simulink model "draft_arm_model"  (R2021b)
settings: Solver=VariableStepAuto  StartTime=0.0  StopTime=8  RelTol=1e-3
values from neighbouring files (symbols this model uses):
  gear_i = 2    [draft_model_variables.m]    (also in linear_model_variables.m = 1)
  ka = km    (= 0.0228)    [draft_model_variables.m]    (also in linear_model_variables.m = 0.0849)
  Kd = 2    [draft_model_variables.m]
  Ki = 0    [draft_model_variables.m]
  km = 22.8*1e-3    (= 0.0228)    [draft_model_variables.m]    (also in linear_model_variables.m = 0.0849)
  Kp = 1    [draft_model_variables.m]
  L = 0.475*1e-3    (= 0.000475)    [draft_model_variables.m]    (also in linear_model_variables.m = 0.000273)
  R = 0.713    [draft_model_variables.m]    (also in linear_model_variables.m = 0.345)
libraries: slpidlib x2
settings Model: Creator=ncamp  LastModifiedBy=Davin

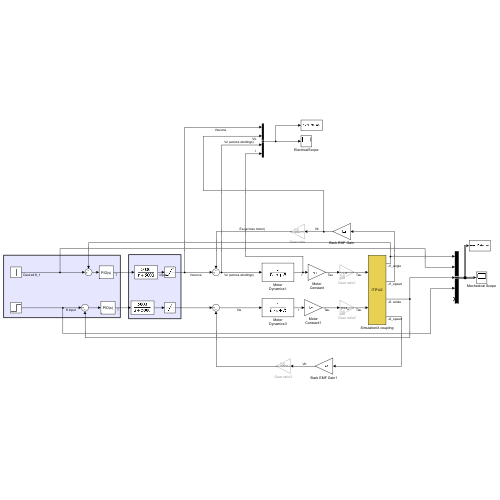
[thumbnail: Simulink's stored preview of the top-level diagram]
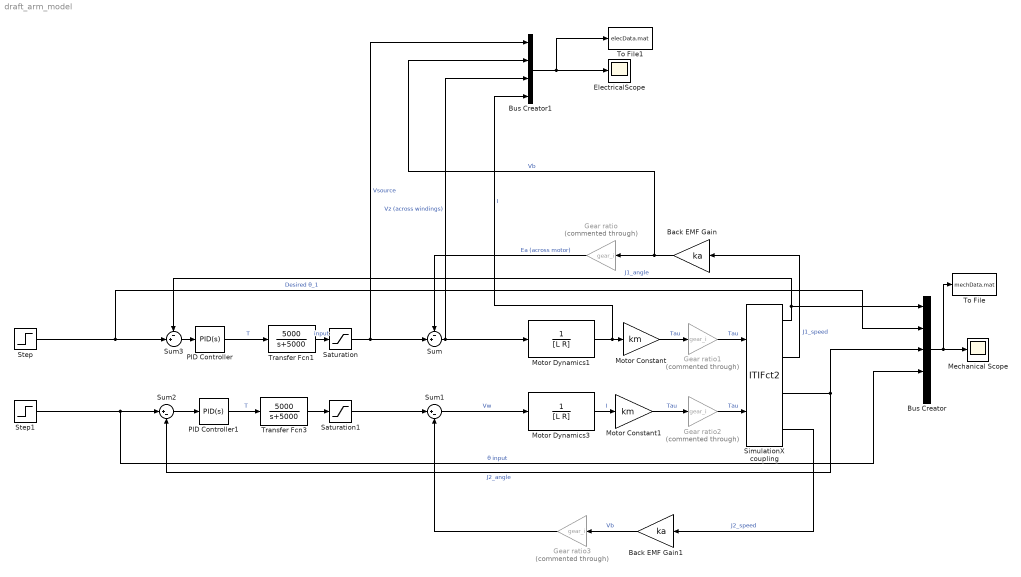
== system draft_arm_model ==
  Back EMF Gain : Gain  Gain=ka
  Back EMF Gain1 : Gain  Gain=ka
  Bus Creator : BusCreator  Inputs=5
  Bus Creator1 : BusCreator  Inputs=4
  ElectricalScope : Scope
  Gear ratio{,1..3} (4 alike) : Gain  Commented=through  Gain=gear_i
  Mechanical Scope : Scope
  Motor Constant : Gain  Gain=km
  Motor Constant1 : Gain  Gain=km
  Motor Dynamics1 : TransferFcn  Denominator=[L R]
  Motor Dynamics3 : TransferFcn  Denominator=[L R]
  PID Controller : slpidlib/PID Controller  Controller=PID  Form=Parallel  TimeDomain=Continuous-time  UseExternalTs=off  SampleTime=-1  IntegratorMethod=Forward Euler  FilterMethod=Forward Euler  ControllerParametersSource=internal  P=Kp  I=Ki  D=Kd  UseFilter=on  N=100  TunerSelectOption=Frequency Response Based  InitialConditionSource=internal  InitialConditionForIntegrator=0  InitialConditionForFilter=0  DifferentiatorICPrevScaledInput=0  ExternalReset=none  TrackingMode=off  Kt=1  LimitOutput=off  SatLimitsSource=internal  UpperSaturationLimit=inf  LowerSaturationLimit=-inf  LinearizeAsGain=on  AntiWindupMode=none  Kb=1  POutMin=[]  POutMax=[]  IOutMin=[]  IOutMax=[]  DOutMin=[]  DOutMax=[]  NOutMin=[]  NOutMax=[]  SumOutMin=[]  SumOutMax=[]  SaturationOutMin=[]  SaturationOutMax=[]  PParamMin=[]  PParamMax=[]  IParamMin=[]  IParamMax=[]  DParamMin=[]  DParamMax=[]  NParamMin=[]  NParamMax=[]  KbParamMin=[]  KbParamMax=[]  KtParamMin=[]  KtParamMax=[]  KbOutMin=[]  KbOutMax=[]  KtOutMin=[]  KtOutMax=[]  IntegratorOutMin=[]  IntegratorOutMax=[]  FilterOutMin=[]  FilterOutMax=[]  SumI1OutMin=[]  SumI1OutMax=[]  SumI2OutMin=[]  SumI2OutMax=[]  SumI3OutMin=[]  SumI3OutMax=[]  SumI4OutMin=[]  SumI4OutMax=[]  SumDOutMin=[]  SumDOutMax=[]  DifferentiatorOutMin=[]  DifferentiatorOutMax=[]  FilterDiffOutCoefMin=[]  FilterDiffOutCoefMax=[]  ReciprocalOutMin=[]  ReciprocalOutMax=[]  SumDenOutMin=[]  SumDenOutMax=[]  SumNumOutMin=[]  SumNumOutMax=[]  DivideOutMin=[]  DivideOutMax=[]  UdiffTsProdOutMin=[]  UdiffTsProdOutMax=[]  NTsProdOutMin=[]  NTsProdOutMax=[]  UintegralTsProdOutMin=[]  UintegralTsProdOutMax=[]  UngainTsProdOutMin=[]  UngainTsProdOutMax=[]  IntegratorContinuousStateAttributes=''  IntegratorStateMustResolveToSignalObject=off  IntegratorRTWStateStorageClass=Auto  FilterContinuousStateAttributes=''  FilterStateMustResolveToSignalObject=off  FilterRTWStateStorageClass=Auto  ParallelPVariant=InternalParameters  IdealPVariant=Disabled  IVariant=InternalParameters  DVariant=InternalParameters  IntegratorVariant=Continuous  SatVariant=Disabled  AWVariant=Passthrough  PCopyVariant=Disabled  TRVariant=Disabled  FdbkBlocksVariant=Forward  IdealPFdbkVariant=Disabled  SatFdbkVariant=Disabled  DerivativeFilterVariant=ContFilter  NVariant=InternalParameters  NCopyVariant=Disabled  FilterICVariant=InternalICsFilter  IntegratorICVariant=InternalICs  ExternalResetVariant=Disabled  TRSumVariant=Passthrough  SumFdbkVariant=Disabled  SumVariant=Sum_PID  TsampFilterVariant=InternalTs  TsampNgainVariant=Passthrough  TsampIntegralVariant=Passthrough  ExternalSaturationOutDataTypeStr=Inherit: Same as second input
  PID Controller1 : slpidlib/PID Controller  Controller=PID  Form=Parallel  TimeDomain=Continuous-time  UseExternalTs=off  SampleTime=-1  IntegratorMethod=Forward Euler  FilterMethod=Forward Euler  ControllerParametersSource=internal  P=Kp  I=Ki  D=Kd  UseFilter=on  N=100  TunerSelectOption=Frequency Response Based  InitialConditionSource=internal  InitialConditionForIntegrator=0  InitialConditionForFilter=0  DifferentiatorICPrevScaledInput=0  ExternalReset=none  TrackingMode=off  Kt=1  LimitOutput=off  SatLimitsSource=internal  UpperSaturationLimit=inf  LowerSaturationLimit=-inf  LinearizeAsGain=on  AntiWindupMode=none  Kb=1  POutMin=[]  POutMax=[]  IOutMin=[]  IOutMax=[]  DOutMin=[]  DOutMax=[]  NOutMin=[]  NOutMax=[]  SumOutMin=[]  SumOutMax=[]  SaturationOutMin=[]  SaturationOutMax=[]  PParamMin=[]  PParamMax=[]  IParamMin=[]  IParamMax=[]  DParamMin=[]  DParamMax=[]  NParamMin=[]  NParamMax=[]  KbParamMin=[]  KbParamMax=[]  KtParamMin=[]  KtParamMax=[]  KbOutMin=[]  KbOutMax=[]  KtOutMin=[]  KtOutMax=[]  IntegratorOutMin=[]  IntegratorOutMax=[]  FilterOutMin=[]  FilterOutMax=[]  SumI1OutMin=[]  SumI1OutMax=[]  SumI2OutMin=[]  SumI2OutMax=[]  SumI3OutMin=[]  SumI3OutMax=[]  SumI4OutMin=[]  SumI4OutMax=[]  SumDOutMin=[]  SumDOutMax=[]  DifferentiatorOutMin=[]  DifferentiatorOutMax=[]  FilterDiffOutCoefMin=[]  FilterDiffOutCoefMax=[]  ReciprocalOutMin=[]  ReciprocalOutMax=[]  SumDenOutMin=[]  SumDenOutMax=[]  SumNumOutMin=[]  SumNumOutMax=[]  DivideOutMin=[]  DivideOutMax=[]  UdiffTsProdOutMin=[]  UdiffTsProdOutMax=[]  NTsProdOutMin=[]  NTsProdOutMax=[]  UintegralTsProdOutMin=[]  UintegralTsProdOutMax=[]  UngainTsProdOutMin=[]  UngainTsProdOutMax=[]  IntegratorContinuousStateAttributes=''  IntegratorStateMustResolveToSignalObject=off  IntegratorRTWStateStorageClass=Auto  FilterContinuousStateAttributes=''  FilterStateMustResolveToSignalObject=off  FilterRTWStateStorageClass=Auto  ParallelPVariant=InternalParameters  IdealPVariant=Disabled  IVariant=InternalParameters  DVariant=InternalParameters  IntegratorVariant=Continuous  SatVariant=Disabled  AWVariant=Passthrough  PCopyVariant=Disabled  TRVariant=Disabled  FdbkBlocksVariant=Forward  IdealPFdbkVariant=Disabled  SatFdbkVariant=Disabled  DerivativeFilterVariant=ContFilter  NVariant=InternalParameters  NCopyVariant=Disabled  FilterICVariant=InternalICsFilter  IntegratorICVariant=InternalICs  ExternalResetVariant=Disabled  TRSumVariant=Passthrough  SumFdbkVariant=Disabled  SumVariant=Sum_PID  TsampFilterVariant=InternalTs  TsampNgainVariant=Passthrough  TsampIntegralVariant=Passthrough  ExternalSaturationOutDataTypeStr=Inherit: Same as second input
  Saturation : Saturate  UpperLimit=24  LowerLimit=-24
  Saturation1 : Saturate  UpperLimit=24  LowerLimit=-24
  SimulationX coupling : S-Function  FunctionName=ITIFct2  Parameters=ip, port, ts, nIn, nOut  SFunctionDeploymentMode=off  EnableBusSupport=off  mask{ip='localhost', port=4097, ts=0.001, nIn=2, nOut=4}
      mask prompts: ip "Address: ip"; port "Port Number: port [-]"; ts "Communication Step Size: ts [s]"; nIn "Input Vector Dimension (to SimulationX): nIn [-]"; nOut "Output Vector Dimension (from SimulationX): nOut [-]"
      mask help: Coupling Element
  Step : Step  Time=0.5  After=pi/2  SampleTime=0
  Step1 : Step  Time=0.5  After=pi/2  SampleTime=0
  Sum : Sum  Inputs=-+|
  Sum1 : Sum  Inputs=|+-
  Sum2 : Sum  Inputs=|+-
  Sum3 : Sum  Inputs=-+|
  To File : ToFile  Filename=mechData.mat  MatrixName=data  SaveFormat=Timeseries
  To File1 : ToFile  Filename=elecData.mat  SaveFormat=Timeseries
  Transfer Fcn1 : TransferFcn  Numerator=[5000]  Denominator=[1, 5000]
  Transfer Fcn3 : TransferFcn  Numerator=[5000]  Denominator=[1, 5000]
  wires:
  Back EMF Gain/1 -> Bus Creator1/2, Gear ratio/1  "Vb"
  Motor Dynamics1/1 -> Bus Creator1/4, Motor Constant/1  "I"
  Sum/1 -> Bus Creator1/3, Motor Dynamics1/1  "Vz (across windings)"
  Back EMF Gain1/1 -> Gear ratio3/1  "Vb"
  Motor Dynamics3/1 -> Motor Constant1/1  "I"
  Sum1/1 -> Motor Dynamics3/1  "Vw"
  Sum2/1 -> PID Controller1/1
  Step1/1 -> Bus Creator/4, Sum2/1  "θ input"
  PID Controller1/1 -> Transfer Fcn3/1  "T"
  Transfer Fcn3/1 -> Saturation1/1
  PID Controller/1 -> Transfer Fcn1/1  "T"
  Step/1 -> Bus Creator/2, Sum3/2  "Desired θ_1"
  Sum3/1 -> PID Controller/1
  Motor Constant1/1 -> Gear ratio2/1  "Tau"
  Gear ratio2/1 -> SimulationX coupling/2  "Tau"
  Motor Constant/1 -> Gear ratio1/1  "Tau"
  Gear ratio1/1 -> SimulationX coupling/1  "Tau"
  Gear ratio3/1 -> Sum1/2
  Gear ratio/1 -> Sum/1  "Ea (across motor)"
  SimulationX coupling/2 -> Back EMF Gain/1  "J1_speed"
  SimulationX coupling/1 -> Sum3/1, Bus Creator/1  "J1_angle"
  SimulationX coupling/4 -> Back EMF Gain1/1  "J2_speed"
  SimulationX coupling/3 -> Bus Creator/3, Sum2/2  "J2_angle"
  Transfer Fcn1/1 -> Saturation/1  "input"
  Saturation/1 -> Bus Creator1/1, Sum/2  "Vsource"
  Saturation1/1 -> Sum1/1
  Bus Creator/1 -> Mechanical Scope/1, To File/1
  Bus Creator1/1 -> To File1/1, ElectricalScope/1
